simulink model "PD_UAV"  (R2025a)
settings: Solver=VariableStepAuto  StartTime=0.0  StopTime=10.0  RelTol=1e-3
libraries: robotcorelib x2
settings Model: Creator=w1262  LastModifiedBy=w1262
settings DataIOCC: ReturnWorkspaceOutputs=off

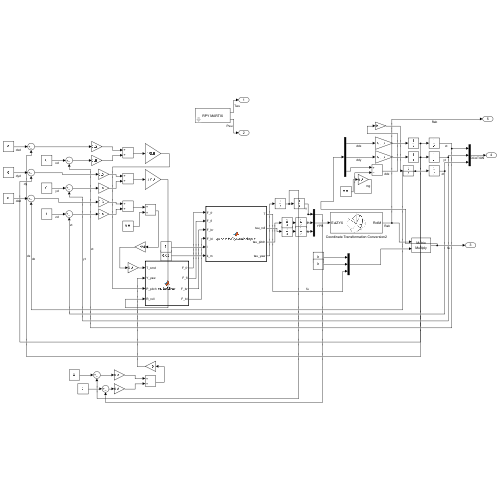
[thumbnail: Simulink's stored preview of the top-level diagram]
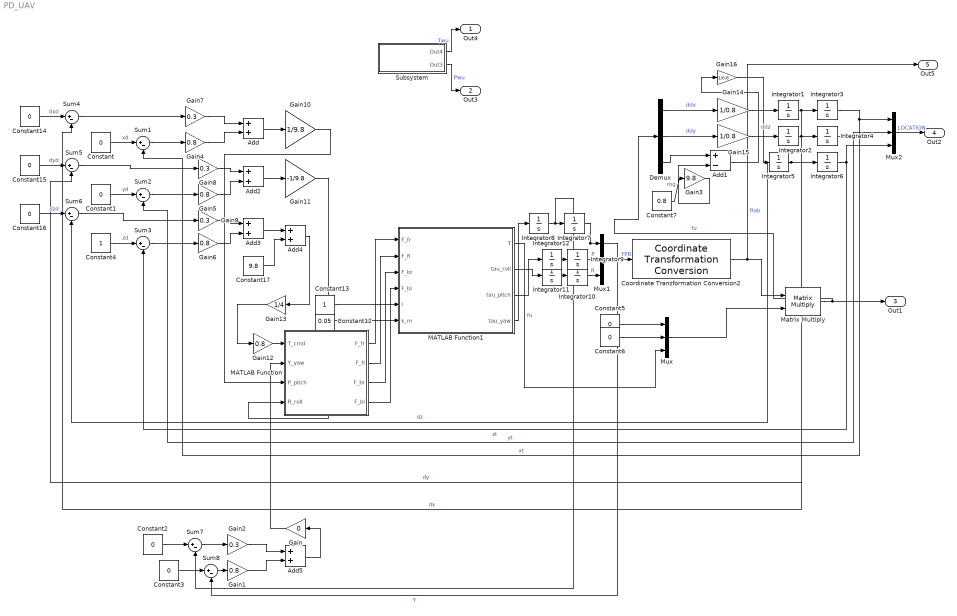
== system PD_UAV ==
  Add{,2..5} (5 alike) : Sum
  Add1 : Sum  Inputs=+-
  Constant{,1..3,5..6,14..16} (9 alike) : Constant  Value=0
  Constant12 : Constant  Value=0.05
  Constant13 : Constant
  Constant17 : Constant  Value=9.8
  Constant4 : Constant
  Constant7 : Constant  Value=0.8
  Coordinate Transformation Conversion2 : robotcorelib/Coordinate Transformation Conversion  InputRepresentation=Euler Angles  InputEulerSequence=ZYX  ShowTrVecInputPort=on  OutputRepresentation=Rotation Matrix  OutputEulerSequence=ZYX  ShowTrVecOutputPort=on  SimulateUsing=Interpreted execution
  Demux : Demux  Outputs=3
  Gain : Gain  Gain=0
  Gain{1,4..6,12} (5 alike) : Gain  Gain=0.8
  Gain10 : Gain  Gain=1/9.8
  Gain11 : Gain  Gain=-1/9.8
  Gain13 : Gain  Gain=1/4
  Gain14 : Gain  Gain=1/0.8
  Gain15 : Gain  Gain=1/0.8
  Gain16 : Gain  Gain=1/0.8
  Gain{2,7..9} (4 alike) : Gain  Gain=0.3
  Gain3 : Gain  Gain=9.8
  Integrator{1..12} (12 alike) : Integrator
  MATLAB Function : MATLAB Function  TreatAsAtomicUnit=on
  MATLAB Function1 : MATLAB Function  TreatAsAtomicUnit=on
  Matrix Multiply : Product  Multiplication=Matrix(*)
  Mux : Mux  Inputs=3
  Mux1 : Mux  Inputs=3
  Mux2 : Mux  Inputs=3
  Subsystem : Subsystem  mask{R=0, P=0, Y=pi/2, x0=3, y0=3, z0=0}
      mask prompts: R "Roll"; P "Pitch"; Y "Yell"; x0 "World X Coordinate"; y0 "World Y Coordinate"; z0 "World Z Coordinate"
      mask DialogControl DescGroupVar Prompt: Input the RPY angel to get the T martix.
      mask DialogControl ParameterGroupVar Prompt: 参数
      mask Display: disp("RPY MARTIX")
  Sum{1..8} (8 alike) : Sum  Inputs=|+-
  Out4 : Outport
  Out3 : Outport  Port=2
  Out1 : Outport  Port=3
  Out2 : Outport  Port=4
  Out5 : Outport  Port=5
  wires:
  Gain1/1 -> Add5/2
  Integrator1/1 -> Integrator3/1, Sum4/2  "dx"
  Add5/1 -> Gain/1
  Constant13/1 -> MATLAB Function1/5(l)
  Constant5/1 -> Mux/1
  Add/1 -> Gain10/1
  Subsystem/2(Out3) -> Out3/1  "Pwu"
  Demux/2 -> Gain15/1  "ddy"
  Constant1/1 -> Sum2/1  "yd"
  Gain8/1 -> Add2/1
  MATLAB Function1/2(tau_roll) -> Integrator11/1
  Mux2/1 -> Out2/1  "LOCATION"
  Integrator9/1 -> Mux1/2  "P"
  MATLAB Function1/3(tau_pitch) -> Integrator12/1
  Integrator10/1 -> Mux1/3  "R"
  Sum1/1 -> Gain4/1
  Sum7/1 -> Gain2/1
  Constant2/1 -> Sum7/1
  Constant15/1 -> Sum5/1  "dyd"
  Demux/3 -> Add1/1
  Gain16/1 -> Integrator5/1
  Integrator6/1 -> Sum3/2, Mux2/3  "zt"
  Demux/1 -> Gain14/1  "ddx"
  Add1/1 -> Gain16/1  "ddz"
  Add3/1 -> Add4/1
  Mux/1 -> Matrix Multiply/2
  Constant16/1 -> Sum6/1  "dzd"
  Constant3/1 -> Sum8/1
  Sum3/1 -> Gain6/1
  Matrix Multiply/1 -> Demux/1, Out1/1  "fu"
  Sum4/1 -> Gain7/1
  Gain6/1 -> Add3/2
  Gain12/1 -> MATLAB Function/1(T_cmd)
  Constant12/1 -> MATLAB Function1/6(k_m)
  Constant17/1 -> Add4/2
  Integrator4/1 -> Sum2/2, Mux2/2  "yt"
  Constant7/1 -> Gain3/1
  Constant14/1 -> Sum4/1  "dxd"
  Sum5/1 -> Gain8/1
  Gain3/1 -> Add1/2  "mg"
  Integrator7/1 -> Sum8/2, Mux1/1  "Y"
  Integrator12/1 -> Integrator9/1
  MATLAB Function/4(F_bl) -> MATLAB Function1/4(F_bl)
  Sum2/1 -> Gain5/1
  Add4/1 -> Gain13/1
  Integrator5/1 -> Sum6/2, Integrator6/1  "dz"
  Gain/1 -> MATLAB Function/2(Y_yaw)
  Integrator3/1 -> Mux2/1, Sum1/2  "xt"
  Sum6/1 -> Gain9/1
  Add2/1 -> Gain11/1
  Constant/1 -> Sum1/1  "xd"
  MATLAB Function/2(F_fl) -> MATLAB Function1/2(F_fl)
  Integrator8/1 -> Sum7/2, Integrator7/1
  Mux1/1 -> Coordinate Transformation Conversion2/1  "YPR"
  Constant4/1 -> Sum3/1  "zd"
  MATLAB Function1/1(T) -> Mux/3  "fu"
  MATLAB Function1/4(tau_yaw) -> Integrator8/1
  Gain5/1 -> Add2/2
  Gain9/1 -> Add3/1
  Gain10/1 -> MATLAB Function/3(P_pitch)
  Gain15/1 -> Integrator2/1
  Sum8/1 -> Gain1/1
  MATLAB Function/3(F_br) -> MATLAB Function1/3(F_br)
  Integrator2/1 -> Integrator4/1, Sum5/2  "dy"
  Gain11/1 -> MATLAB Function/4(R_roll)
  Integrator11/1 -> Integrator10/1
  Subsystem/1(Out4) -> Out4/1  "Twu"
  Gain2/1 -> Add5/1
  Coordinate Transformation Conversion2/1 -> Matrix Multiply/1, Out5/1  "Rab"
  Constant6/1 -> Mux/2
  Gain13/1 -> Gain12/1
  Gain4/1 -> Add/2
  Gain14/1 -> Integrator1/1
  Gain7/1 -> Add/1
  MATLAB Function/1(F_fr) -> MATLAB Function1/1(F_fr)

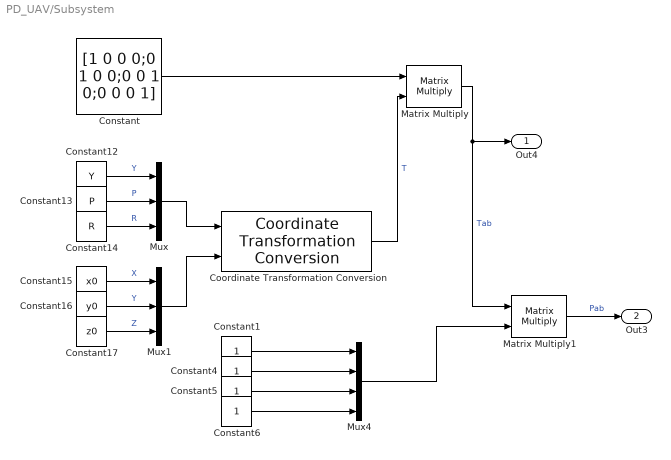
== system PD_UAV/Subsystem ==
  Constant : Constant  Value=[1 0 0 0;0 1 0 0;0 0 1 0;0 0 0 1]
  Constant{1,4..6} (4 alike) : Constant
  Constant12 : Constant  Value=Y
  Constant13 : Constant  Value=P
  Constant14 : Constant  Value=R
  Constant15 : Constant  Value=x0
  Constant16 : Constant  Value=y0
  Constant17 : Constant  Value=z0
  Coordinate Transformation Conversion : robotcorelib/Coordinate Transformation Conversion  InputRepresentation=Euler Angles  InputEulerSequence=ZYX  ShowTrVecInputPort=on  OutputRepresentation=Homogeneous Transformation  OutputEulerSequence=ZYX  ShowTrVecOutputPort=on  SimulateUsing=Interpreted execution
  Matrix Multiply : Product  Multiplication=Matrix(*)
  Matrix Multiply1 : Product  Multiplication=Matrix(*)
  Mux : Mux  Inputs=3
  Mux1 : Mux  Inputs=3
  Mux4 : Mux
  Out4 : Outport
  Out3 : Outport  Port=2
  wires:
  Mux1/1 -> Coordinate Transformation Conversion/2
  Constant12/1 -> Mux/1  "Y"
  Constant16/1 -> Mux1/2  "Y"
  Mux/1 -> Coordinate Transformation Conversion/1
  Matrix Multiply/1 -> Out4/1, Matrix Multiply1/1  "Tab"
  Constant/1 -> Matrix Multiply/1
  Coordinate Transformation Conversion/1 -> Matrix Multiply/2  "T"
  Constant14/1 -> Mux/3  "R"
  Matrix Multiply1/1 -> Out3/1  "Pab"
  Constant15/1 -> Mux1/1  "X"
  Constant13/1 -> Mux/2  "P"
  Constant6/1 -> Mux4/4
  Constant1/1 -> Mux4/1
  Constant4/1 -> Mux4/2
  Constant5/1 -> Mux4/3
  Constant17/1 -> Mux1/3  "Z"
  Mux4/1 -> Matrix Multiply1/2

== matlab function PD_UAV/MATLAB Function1 ==
  data: F_fr input; T output; F_fl input; F_br input; F_bl input; tau_roll output; tau_pitch output; tau_yaw output; l input; k_m input
function [T, tau_roll, tau_pitch, tau_yaw] = ...
    quadrotorDynamicsInput( ...
    F_fr, F_fl, F_br, F_bl, l, k_m)

% quadrotorDynamicsInput
% 四旋翼推力与控制力矩计算函数
%
% 输入：
% F_fr : 前右旋翼推力
% F_fl : 前左旋翼推力
% F_br : 后右旋翼推力
% F_bl : 后左旋翼推力
%
% l    : 旋翼到机体质心距离
% k_m  : 偏航力矩系数
%
% 输出：
% T          : 总推力
% tau_phi    : Roll 力矩
% tau_theta  : Pitch 力矩
% tau_psi    : Yaw 力矩

%% 总推力
T = F_fl + F_fr + F_bl + F_br;
%% Roll 力矩 (绕 x_u 轴)
tau_roll = ...
    l * ( ...
    F_fr + F_br ...
    - F_fl - F_bl ...
    );
%% Pitch 力矩 (绕 y_u 轴)
tau_pitch = ...
    l * ( ...
    F_bl + F_br ...
    - F_fl - F_fr ...
    );
%% Yaw 力矩 (绕 z_u 轴)
tau_yaw = ...
    k_m * ( ...
    F_fl - F_fr ...
    - F_bl + F_br ...
    );
end

== matlab function PD_UAV/MATLAB Function ==
  data: T_cmd input; F_fr output; Y_yaw input; P_pitch input; R_roll input; F_fl output; F_br output; F_bl output
function [F_fr, F_fl, F_br, F_bl] = motorMixer( ...
    T_cmd, Y_yaw, P_pitch, R_roll)

% motorMixer
% 四旋翼控制分配函数（Motor Mixer）

F_fr = T_cmd + Y_yaw + P_pitch + R_roll;
F_fl = T_cmd - Y_yaw + P_pitch - R_roll;
F_br = T_cmd - Y_yaw - P_pitch + R_roll;
F_bl = T_cmd + Y_yaw - P_pitch - R_roll;

end
